simulink model "pid_controller"  (R2023b)
settings: Solver=FixedStepDiscrete  StartTime=0.0  StopTime=10.0  RelTol=1e-3
values from neighbouring files (symbols this model uses):
  kc_1 = 1    [ca2_params.m]    (also in iterate_gains.m = 0.5)
  kI_1 = 1    [ca2_params.m]    (also in iterate_gains.m = 0.01)
undefined symbols (not defined in the file or in its folder): DiscIntNeverNeededParam
settings Model: Creator=john  LastModifiedBy=john

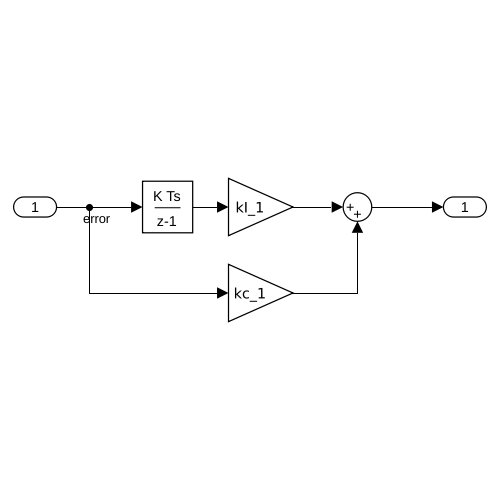
[thumbnail: Simulink's stored preview of the top-level diagram]
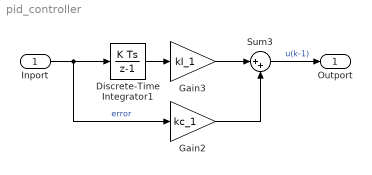
== system pid_controller ==
  Inport : Inport
  Discrete-Time Integrator1 : DiscreteIntegrator  SampleTime=-1  ICPrevOutput=DiscIntNeverNeededParam  ICPrevScaledInput=DiscIntNeverNeededParam
  Gain2 : Gain  Gain=kc_1
  Gain3 : Gain  Gain=kI_1
  Sum3 : Sum  Inputs=|++
  Outport : Outport
  wires:
  Inport/1 -> Gain2/1, Discrete-Time Integrator1/1  "error"
  Sum3/1 -> Outport/1  "u(k-1)"
  Discrete-Time Integrator1/1 -> Gain3/1
  Gain3/1 -> Sum3/1
  Gain2/1 -> Sum3/2
